simulink model "common_blocks"  (Simulink 8.9)
settings: Solver=ode45  StartTime=0.0  StopTime=0.3  RelTol=1e-3  EnableMultiTasking=on
settings Model: Creator=tnichols  LastModifiedBy=mbodson
settings SolverCC: ZeroCrossControl=DisableAll
settings DataIOCC: LimitDataPoints=off  TimeSaveName=t
settings OptimizationCC: ExpressionDepthLimit=2147483647
settings ConfigComp: CovSFcnEnable=off

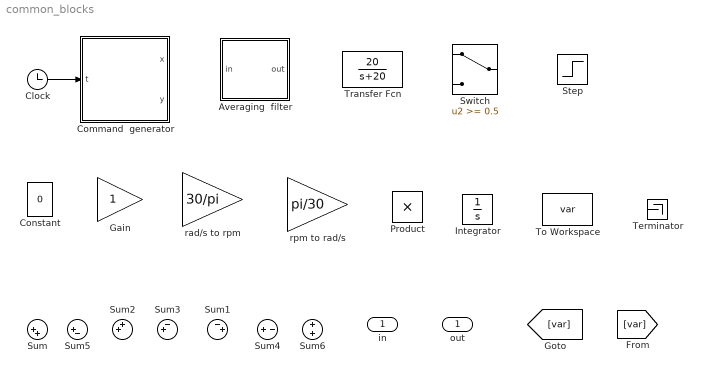
== system common_blocks ==
  in : Inport
  Averaging  filter : Subsystem
  Clock : Clock
  Command  generator : MATLAB Function  TreatAsAtomicUnit=on
  Constant : Constant  Value=0
  Gain : Gain
  Integrator : Integrator
  Product : Product  RndMeth=Zero
  Step : Step  Time=0.1  After=10  SampleTime=0
  Sum : Sum  Inputs=|++
  Sum1 : Sum  Inputs=-+|
  Sum2 : Sum  Inputs=++|
  Sum3 : Sum  Inputs=-+|
  Sum4 : Sum  Inputs=+|-
  Sum5 : Sum  Inputs=|+-
  Sum6 : Sum
  Switch : Switch  Threshold=0.5
  Terminator : Terminator
  To Workspace : ToWorkspace  VariableName=var  SampleTime=-1
  Transfer Fcn : TransferFcn  Numerator=[20]  Denominator=[1 20]
  rad/s to rpm : Gain  Gain=30/pi
  rpm to rad/s : Gain  Gain=pi/30
  out : Outport
  wires:
  Clock/1 -> Command  generator/1(t)

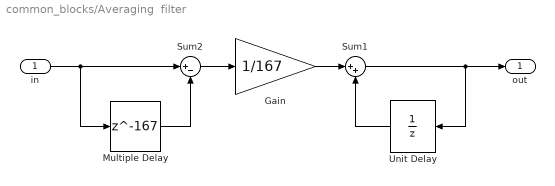
== system common_blocks/Averaging  filter ==
  in : Inport
  Gain : Gain  Gain=1/167  SaturateOnIntegerOverflow=on  OutDataTypeStr=Inherit: Same as input  ParamDataTypeStr=Inherit: Same as input
  Multiple Delay : Delay  DelayLength=167  InitialCondition=0  InputProcessing=Inherited  SampleTime=1e-4
  Sum1 : Sum  Inputs=|++
  Sum2 : Sum  Inputs=|+-
  Unit Delay : UnitDelay  SampleTime=1e-4
  out : Outport
  wires:
  Sum2/1 -> Gain/1
  in/1 -> Sum2/1, Multiple Delay/1
  Sum1/1 -> out/1, Unit Delay/1
  Gain/1 -> Sum1/1
  Unit Delay/1 -> Sum1/2
  Multiple Delay/1 -> Sum2/2

== matlab function Command generator ==
  data: t input double size=1; x output double; y output double
function [x,y]  = CG(t)
x=0;y=0;
if t>1
    x=1;
    y=3;
end
